simulink model "MCLV2_dsPIC33EP256MC506_externalOpAmp_CurrentLoop_FrSky"  (R2019a)
settings: Solver=FixedStepDiscrete  StartTime=0.0  StopTime=inf  FixedStep=.00005  RelTol=1e-3  EnableMultiTasking=on
values from neighbouring files (symbols this model uses):
  Imax = Inom    (= 4.3)    [DCMotorParameters.m]
  Imin = -Inom    (= -4.3)    [DCMotorParameters.m]
  Ke = place(Ae,Be,Elec_desired_poles)    [DCMotorParameters.m]
  Km = place(Am,Bm,Desired_mecha_pole)    [DCMotorParameters.m]
  Ommax = Omnom    (= 350)    [DCMotorParameters.m]
  Ommin = -Omnom    (= -350)    [DCMotorParameters.m]
  Ts = 0.5e-4    (= 5e-05)    [DCMotorParameters.m]
  TsMeca = 0.002    [DCMotorParameters.m]
  Vmax = Vdc    (= 24)    [DCMotorParameters.m]
  Vmin = -Vdc    (= -24)    [DCMotorParameters.m]
undefined symbols (not defined in the file or in its folder): A4, A8, B5, B6, C10, C5, C6, D5, DiscIntNeverNeededParam, F0, F1, Max, ms, NumBits1, NumBits2, P20, P24, P37, P53, P54, P97, Pin, PWMmax, Resol, us
libraries: simulink x26, MCHP_Blockset x25, UxV_Blockset x4
(part 2 of 2)

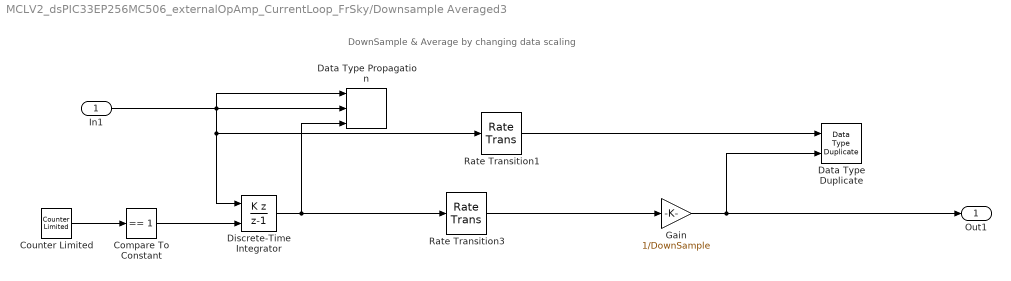
== system MCLV2_dsPIC33EP256MC506_externalOpAmp_CurrentLoop_FrSky/Downsample Averaged3 ==
  note: DownSample & Average by changing data scaling
  In1 : Inport
  Compare To Constant : simulink/Logic and Bit Operations/Compare To Constant  relop===  const=1  OutDataTypeStr=boolean
  Counter Limited : simulink/Sources/Counter Limited  uplimit=DownSample-1  tsamp=-1
  Data Type Duplicate : DataTypeDuplicate
  Data Type Propagation : simulink/Signal Attributes/Data Type Propagation  PropDataType=fixdt(1, 16)  IfRefDouble=double  IfRefSingle=single  IsSigned=IsSigned1 or IsSigned2  NumBitsBase=NumBits1+NumBits2  NumBitsMult=1  NumBitsAdd=0  NumBitsAllowFinal=1:128  PropScaling=2^-10  ValuesUsedBestPrec=[5 -7]  SlopeBase=Slope1  SlopeMult=1  SlopeAdd=0  BiasBase=Bias1  BiasMult=1  BiasAdd=0
      settings: SourceProductName=Simulink  SourceProductBaseCode=SL
  Discrete-Time Integrator : DiscreteIntegrator  IntegratorMethod=Accumulation: Backward Euler  gainval=1  ExternalReset=sampled level  SampleTime=-1  OutDataTypeStr=Inherit: Inherit via back propagation  ICPrevOutput=DiscIntNeverNeededParam  ICPrevScaledInput=DiscIntNeverNeededParam
  Gain : Gain  Gain=1/DownSample  OutDataTypeStr=Inherit: Inherit via back propagation
  Rate Transition1 : RateTransition  Deterministic=off  OutPortSampleTime=[InputSampleTime * DownSample]
  Rate Transition3 : RateTransition  OutPortSampleTime=[InputSampleTime * DownSample]
  Out1 : Outport
  wires:
  Rate Transition3/1 -> Gain/1
  In1/1 -> Discrete-Time Integrator/1, Rate Transition1/1, Data Type Propagation/2, Data Type Propagation/1
  Compare To Constant/1 -> Discrete-Time Integrator/2
  Discrete-Time Integrator/1 -> Data Type Propagation/3, Rate Transition3/1
  Counter Limited/1 -> Compare To Constant/1
  Gain/1 -> Data Type Duplicate/2, Out1/1
  Rate Transition1/1 -> Data Type Duplicate/1

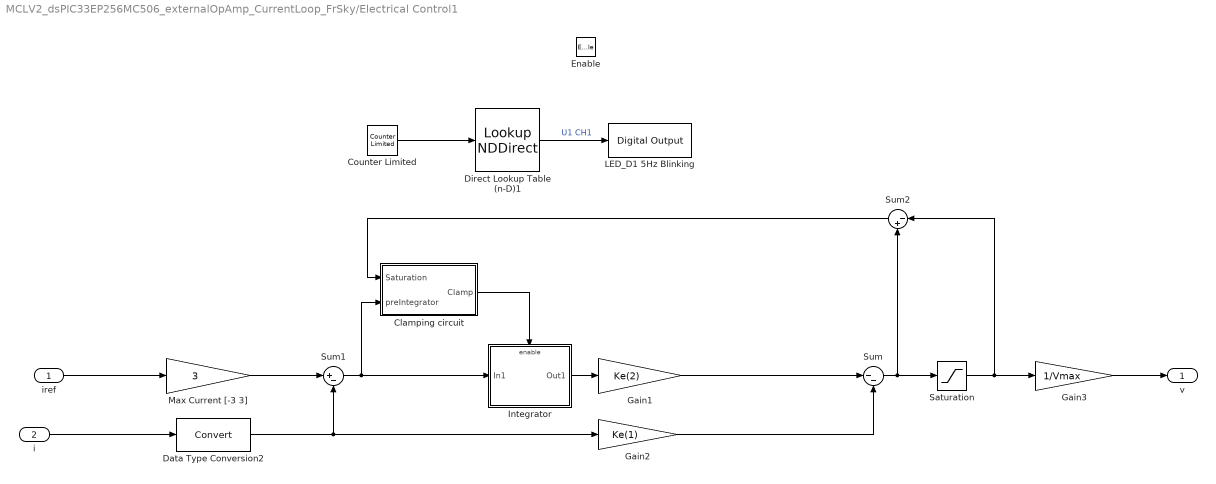
== system MCLV2_dsPIC33EP256MC506_externalOpAmp_CurrentLoop_FrSky/Electrical Control1 ==
  iref : Inport
  i : Inport  Port=2
  Enable : EnablePort  StatesWhenEnabling=reset
  Clamping circuit : Subsystem
  Counter Limited : simulink/Sources/Counter Limited  uplimit=9  tsamp=.1
  Data Type Conversion2 : DataTypeConversion  SaturateOnIntegerOverflow=on
  Direct Lookup Table (n-D)1 : LookupNDDirect  NumberOfTableDimensions=1  Table=[1 0 0 0 0 0 0 0 0 0]  TableDataTypeStr=boolean
  Gain1 : Gain  Gain=Ke(2)  OutMin=[2*Vmin]  OutMax=[2*Vmax]  OutDataTypeStr=fixdt(1,16)
  Gain2 : Gain  Gain=Ke(1)  OutMin=[2*Vmin]  OutMax=[2*Vmax]  OutDataTypeStr=fixdt(1,16)
  Gain3 : Gain  Gain=1/Vmax  OutDataTypeStr=fixdt(1,16,15)  SaturateOnIntegerOverflow=on
  Integrator : Subsystem
  LED_D1 5Hz Blinking : MCHP_Blockset/Digital IO/Digital Output  PORT=Dynamic Options  PORT_TXT="D   [ 5  6  8 ]"  PIN=6  PACK=off  SIMULTANEOUS=off  READPREVIOUS=off  ORDERING=None  SampleTime=-1  MCHP_MASTERLINK=MCLV2_dsPIC33EP256MC506_externalOpAmp_CurrentLoop_FrSky/Microchip Master
      settings: SourceProductName=MPLAB Device Blocks for Simulink
  Max Current [-3 3] : Gain  Gain=3  OutMin=-3  OutMax=3  OutDataTypeStr=fixdt(1,16)
  Saturation : Saturate  UpperLimit=Vmax  LowerLimit=Vmin
  Sum : Sum  Inputs=|--  SaturateOnIntegerOverflow=on
  Sum1 : Sum  Inputs=|+-  OutMin=[2*Imin]  OutMax=[2*Imax]  OutDataTypeStr=fixdt(1,16)  SaturateOnIntegerOverflow=on
  Sum2 : Sum  Inputs=|-+  OutDataTypeStr=Inherit: Same as accumulator
  v : Outport
  wires:
  iref/1 -> Max Current [-3 3]/1
  i/1 -> Data Type Conversion2/1
  Gain1/1 -> Sum/1
  Gain2/1 -> Sum/2
  Saturation/1 -> Sum2/1, Gain3/1
  Sum1/1 -> Integrator/1(In1), Clamping circuit/2(preIntegrator)
  Integrator/1(Out1) -> Gain1/1
  Clamping circuit/1(Clamp) -> Integrator/Enable
  Sum/1 -> Saturation/1, Sum2/2
  Sum2/1 -> Clamping circuit/1(Saturation)
  Data Type Conversion2/1 -> Gain2/1, Sum1/2
  Gain3/1 -> v/1
  Max Current [-3 3]/1 -> Sum1/1
  Direct Lookup Table (n-D)1/1 -> LED_D1 5Hz Blinking/1  "U1 CH1"
  Counter Limited/1 -> Direct Lookup Table (n-D)1/1

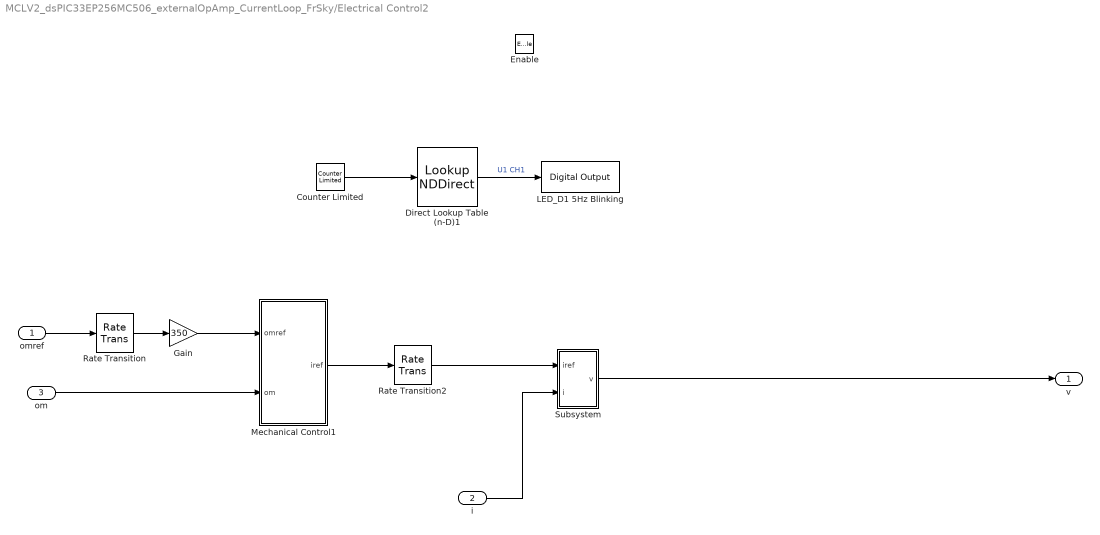
== system MCLV2_dsPIC33EP256MC506_externalOpAmp_CurrentLoop_FrSky/Electrical Control2 ==
  omref : Inport
  i : Inport  Port=2
  om : Inport  Port=3
  Enable : EnablePort  StatesWhenEnabling=reset
  Counter Limited : simulink/Sources/Counter Limited  uplimit=9  tsamp=.1
  Direct Lookup Table (n-D)1 : LookupNDDirect  NumberOfTableDimensions=1  Table=[1 0 1 0 0 0 0 0 0 0]  TableDataTypeStr=boolean
  Gain : Gain  Gain=350  OutDataTypeStr=Inherit: Inherit via back propagation
  LED_D1 5Hz Blinking : MCHP_Blockset/Digital IO/Digital Output  PORT=Dynamic Options  PORT_TXT="D   [ 5  6  8 ]"  PIN=6  PACK=off  SIMULTANEOUS=off  READPREVIOUS=off  ORDERING=None  SampleTime=-1  MCHP_MASTERLINK=MCLV2_dsPIC33EP256MC506_externalOpAmp_CurrentLoop_FrSky/Microchip Master
      settings: SourceProductName=MPLAB Device Blocks for Simulink
  Mechanical Control1 : Subsystem
  Rate Transition : RateTransition  Deterministic=off
  Rate Transition2 : RateTransition  Deterministic=off
  Subsystem : Subsystem
  v : Outport
  wires:
  i/1 -> Subsystem/2(i)
  Subsystem/1(v) -> v/1
  Mechanical Control1/1(iref) -> Rate Transition2/1
  Rate Transition2/1 -> Subsystem/1(iref)
  omref/1 -> Rate Transition/1
  Gain/1 -> Mechanical Control1/1(omref)
  Rate Transition/1 -> Gain/1
  om/1 -> Mechanical Control1/2(om)
  Direct Lookup Table (n-D)1/1 -> LED_D1 5Hz Blinking/1  "U1 CH1"
  Counter Limited/1 -> Direct Lookup Table (n-D)1/1

== system MCLV2_dsPIC33EP256MC506_externalOpAmp_CurrentLoop_FrSky/From Pot ==
  In1 : Inport
  Enable : EnablePort
  Cast5 : DataTypeConversion  OutDataTypeStr=boolean
  Counter Free-Running : simulink/Sources/Counter Free-Running  NumBits=1  tsamp=.1
  Gain : Gain  OutDataTypeStr=fixdt(1,16,15)
  LED_D1 5Hz Blinking : MCHP_Blockset/Digital IO/Digital Output  PORT=Dynamic Options  PORT_TXT="D   [ 5  6  8 ]"  PIN=6  PACK=off  SIMULTANEOUS=off  READPREVIOUS=off  ORDERING=None  SampleTime=-1  MCHP_MASTERLINK=MCLV2_dsPIC33EP256MC506_externalOpAmp_CurrentLoop_FrSky/Microchip Master
      settings: SourceProductName=MPLAB Device Blocks for Simulink
  Out1 : Outport
  wires:
  In1/1 -> Gain/1
  Gain/1 -> Out1/1  "Duty Cycle"
  Cast5/1 -> LED_D1 5Hz Blinking/1  "U1 CH1"
  Counter Free-Running/1 -> Cast5/1

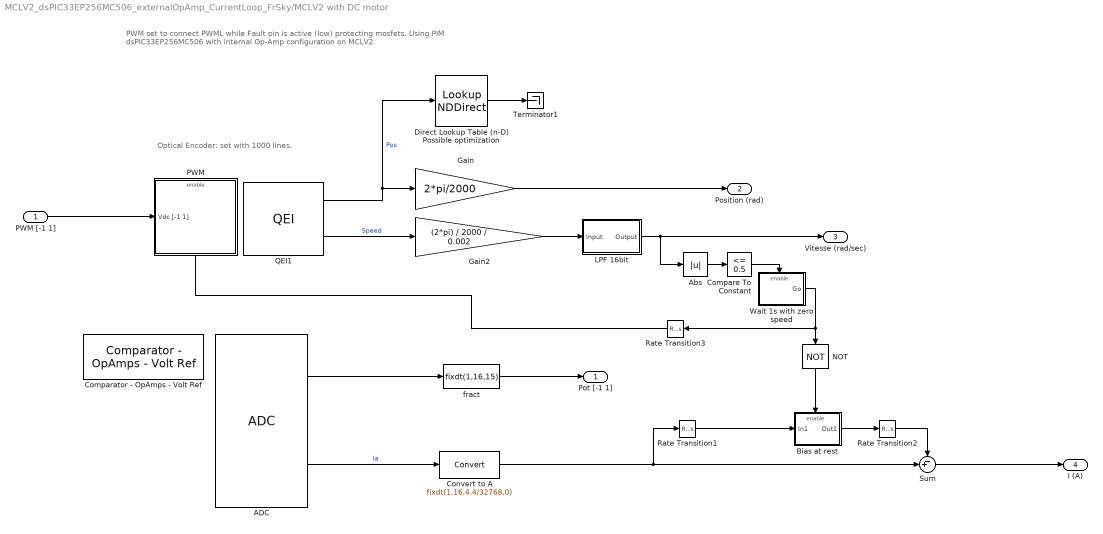
== system MCLV2_dsPIC33EP256MC506_externalOpAmp_CurrentLoop_FrSky/MCLV2 with DC motor ==
  note: PWM set to connect PWML while Fault pin is active (low) protecting mosfets.
      | Using PIM dsPIC33EP256MC506 with internal Op-Amp configuration on MCLV2
  note: Optical Encoder: set with 1000 lines.
  PWM [-1 1] : Inport
  ADC : MCHP_Blockset/Analog IO/ADC  Priority=5  ADC_REF=1  Mode=10 bits (allows exact simultaneous sampling)  FORM="sddd dddd dddd 0000  ==> Signed fractional"  ADC_R="< 5    kOhm"  nSAMPLECHANNELS=CH0 : CH1  nSAMPLECHANNELS_12bits=CH0 only  SIMULTANEOUS=Simultaneously on all Channels  ADxCSS=[13]  MUXA_CH0N=off  MUXA_CH123=Dynamic Options  MUXA_CH123_TXT=OA2 : AN1 : AN2  MUXB_CH0=AN1  MUXB_CH0N=on  MUXB_CH123=Dynamic Options  MUXB_CH123_TXT=OA2 : AN1 : AN2  SequenceRepeat=1  SequenceTiming=are done as fast as possible ; triggered by user define source  SSRC_SSRCG=Dynamic Options  SSRC_SSRCG_TXT=6  Update_BlockOutput=After each trig and conversion sequence  Trig_TimeStep=with each update of the ADC block output  ADC_DMA_CHANNEL=Use Interrupt instead of DMA  SampleTime=5e-05  Info=Total Time for Sample & Conversion : 2.4e-06s including 3.4286e-07s (x 1) sample time.  MCHP_PORT={Analog Input 0}{AN0}15:2:A0;{Analog Input 13}{AN13}15:2:E13;  MCHP_MASTERLINK=MCLV2_dsPIC33EP256MC506_externalOpAmp_CurrentLoop_FrSky/Microchip Master  ADC_TIMING=[2.4000000000000003149e-06]
      settings: SourceProductName=MPLAB Device Blocks for Simulink
  Abs : Abs
  Bias at rest : Subsystem  TreatAsAtomicUnit=on
  Comparator - OpAmps - Volt Ref : MCHP_Blockset/Analog IO/Comparator - OpAmps - Volt Ref  MCHP_params=s.CVR1OE=0;s.CVR2OE=0;s.VREFSEL=0;s.RLaddle=reshape([1 1],1,2);s.AVdd=reshape({ '3.3','3.3'},1,2);s.AVss=reshape({ '0','0'},1,2);s.CVRSS=reshape([0 0],1,2);s.CON_OPMODE_CPOL=reshape([0 3 0 0 0],1,5);s.OutputPort_COE_RP=reshape({ 'B1 / Pin[16] / OA1OUT / AN3 / OA1OUT','A0 / Pin[13] / OA2OUT / AN0 / OA2OUT','C0 / Pin[21] / OA3OUT / AN6 / OA3OUT','None','None'},1,5);s.InputP_CREF=reshape([0 0 0 0 0],1,5);s.InputN_CCH=reshape([0 0 0 0 0],1,5);s.Trigger_EventInterrupt_EVPOL=reshape([0 0 0 0 0],1,5);s.BlockOutputEvent=reshape([0 0 0 0 0],1,5);s.BlockOutputState=reshape([0 0 0 0 0],1,5);s.IntPriority=5;s.FilterFreq=reshape([1e+10 1e+10 1e+10 1e+10 1e+10],1,5);s.Blanking=reshape([1 1 1 1 1],1,5);s.BlankingSignal=reshape({ ' - ',' - ',' - ',' - ',' - ',' - ',' - ',' - ',' - ',' - ',' - ',' - ',' - ',' - ',' - '},3,5);s.BlankingTruthTable=reshape([-1 -1 -1 -1 -1 -1 -1 -1 -1 -1 -1 -1 -1 -1 -1 -1 -1 -1 -1 -1 -1 -1 -1 -1 -1 -1 -1 -1 -1 -1 -1 -1 -1 -1 -1 -1 -1 -1 -1 -1 -1 -1 -1 -1 -1 -1 -1 -1 -1 -1 -1 -1 -1 -1 -1 -1 -1 -1 -1 -1 -1 -1 -1 -1 -1 -1 -1 -1 -1 -1 -1 -1 -1 -1 -1 -1 -1 -1 -1 -1 -1 -1 -1 -1 -1 -1 -1 -1 -1 -1 -1 -1 -1 -1 -1 -1 -1 -1 -1 -1 -1 -1 -1 -1 -1 -1 -1 -1 -1 -1 -1 -1 -1 -1 -1 -1 -1 -1 -1 -1 -1 -1 -1 -1 -1 -1 -1 -1 -1 -1 -1 -1 -1 -1 -1 -1 -1 -1 -1 -1 -1 -1 -1 -1 -1 -1 -1 -1 -1 -1 -1 -1 -1 -1 -1 -1 -1 -1 -1 -1 -1 -1 -1 -1 -1 -1 -1 -1 -1 -1 -1 -1 -1 -1 -1 -1 -1 -1 -1 -1 -1 -1 -1 -1 -1 -1 -1 -1 -1 -1 -1 -1 -1 -1 -1 -1 -1 -1 -1 -1 -1 -1 -1 -1 -1 -1 -1 -1 -1 -1 -1 -1 -1 -1 -1 -1 -1 -1 -1 -1 -1 -1 -1 -1 -1 -1 -1 -1 -1 -1 -1 -1 -1 -1 -1 -1 -1 -1 -1 -1],16 ,3 ,5);  S_INPUT="[5  5]"  S_OUTPUT=[5]  S_INPUT_Size="[2  2]"  S_OUTPUT_Size=[4]  SampleTime=-1  MCHP_MASTERLINK=MCLV2_dsPIC33EP256MC506_externalOpAmp_CurrentLoop_FrSky/Microchip Master  MCHP_PORT={Op-Amp Output 2}{OA2(out)}14:2:A0;{Op-Amp2 V+}{OA2 V+}14:2:A1;{Op-Amp2 V-}{OA2 V-}14:2:B0;  ORDERING=0
      settings: SourceProductName=MPLAB Device Blocks for Simulink
  Compare To Constant : simulink/Logic and Bit Operations/Compare To Constant  relop=<=  const=0.5  OutDataTypeStr=boolean
  Convert to A : DataTypeConversion  OutDataTypeStr=fixdt(1,16,4.4/32768,0)  ConvertRealWorld=Stored Integer (SI)
  Direct Lookup Table (n-D) Possible optimization : LookupNDDirect  NumberOfTableDimensions=1  Table=[0:(1000-1)]*2*pi/1000  TableDataTypeStr=fixdt(1,16,5)
      settings: LockScale=on
  Gain : Gain  Gain=2*pi/2000  OutDataTypeStr=fixdt(1,16,5)
  Gain2 : Gain  Gain=(2*pi) / 2000 / 0.002  OutDataTypeStr=fixdt(1,16,5)  LockScale=on
  "LPF 16bit " : Subsystem  Tag=FilterWizardSubSystem
      settings: ErrorFcn=dspFilterRealizedInBasicElemsAlgLoopErrFcnCallback
  NOT : Logic  Operator=NOT  IconShape=distinctive  AllPortsSameDT=off  OutDataTypeStr=boolean
  PWM : Subsystem
  QEI1 : MCHP_Blockset/QEI/QEI  QEI_REF=1  QEI_MODE=Quadrature Encoder  QEI_x2mode=off  QEI_PulseCountDir=Down  PIN_QEA=Dynamic Options  PIN_QEA_TXT=A8 / P24 / Pin[31]  PIN_QEB=Dynamic Options  PIN_QEB_TXT=C6 / P54 / Pin[50]  SWPAB=off  QEAPOL=off  QEBPOL=off  SampleTime=.002  PIN_CCMP=Dynamic Options  PIN_CCMP_TXT=A4 / P20 / Pin[33]  MCHP_PORT={QEI1 A}{QEIA1}5:0:P24;{QEI1 B}{QEIB1}5:0:P54;  MCHP_MASTERLINK=MCLV2_dsPIC33EP256MC506_externalOpAmp_CurrentLoop_FrSky/Microchip Master  INDXxCNT_Output=is not an output  POSxCNT_Output=is a 16 bits unsigned block output  RESET_Input=off  PIMOD_mode=position is cyclique between user defined boundaries  PIMOD_modeB=Never reset position  PIMOD_reset=on next INDEX event  PIN_INDEX=Dynamic Options  PIN_INDEX_TXT=A4 / P20 / Pin[33]  IMV=QEA = 1 and QEB = 0  IMV_x2=QEA = 1  PIN_HOME=Dynamic Options  PIN_HOME_TXT=A4 / P20 / Pin[33]  QEIxLEC_GEC=[0 1999]  QEIxIC=0  PCIIRQ=off  IDXPOL=off  HOMPOL=on  VELxCNT_Output=is a 16 bits signed block output  INTxHLD_Output=is not an output  MaxPeriod=1e-3  FILTREN=on  QFDIV_popup=Dynamic Options  QFDIV_popup_TXT=729.17 kHz  FILTER_CutOffFreq=100e3  QEI_IntPri=5
      settings: SourceProductName=MPLAB Device Blocks for Simulink
  Rate Transition1 : RateTransition  Deterministic=off  OutPortSampleTime=.002
  Rate Transition2 : RateTransition  Deterministic=off
  Rate Transition3 : RateTransition  Deterministic=off
  Sum : Sum  Inputs=-+|  OutDataTypeStr=Inherit: Inherit via back propagation  SaturateOnIntegerOverflow=on  InputSameDT=on
  Terminator1 : Terminator
  Wait 1s with zero speed : Subsystem  TreatAsAtomicUnit=on
  fract : DataTypeConversion  OutDataTypeStr=fixdt(1,16,15)  ConvertRealWorld=Stored Integer (SI)
  Pot [-1 1] : Outport
  Position (rad) : Outport  Port=2
  Vitesse (rad/sec) : Outport  Port=3
  I (A) : Outport  Port=4
  wires:
  Abs/1 -> Compare To Constant/1
  Rate Transition3/1 -> PWM/Enable
  Compare To Constant/1 -> Wait 1s with zero speed/Enable
  Wait 1s with zero speed/1(Go) -> NOT/1, Rate Transition3/1
  PWM [-1 1]/1 -> PWM/1(Vdc [-1 1])
  NOT/1 -> Bias at rest/Enable
  Rate Transition2/1 -> Sum/1
  Rate Transition1/1 -> Bias at rest/1(In1)
  Bias at rest/1(Out1) -> Rate Transition2/1
  Sum/1 -> I (A)/1
  ADC/2 -> Convert to A/1  "Ia"
  Convert to A/1 -> Rate Transition1/1, Sum/2
  "LPF 16bit "/1(Output) -> Abs/1, Vitesse (rad/sec)/1
  Gain2/1 -> "LPF 16bit "/1(Input)
  Gain/1 -> Position (rad)/1
  fract/1 -> Pot [-1 1]/1
  QEI1/1 -> Gain/1, Direct Lookup Table (n-D) Possible optimization/1  "Pos"
  ADC/1 -> fract/1
  QEI1/2 -> Gain2/1  "Speed"
  Direct Lookup Table (n-D) Possible optimization/1 -> Terminator1/1

== system MCLV2_dsPIC33EP256MC506_externalOpAmp_CurrentLoop_FrSky/Steps Large ==
  Enable : EnablePort  StatesWhenEnabling=reset
  Constant : Constant  Value=0  OutDataTypeStr=Inherit: Inherit via back propagation
  Counter Limited : simulink/Sources/Counter Limited  uplimit=9  tsamp=.1
  Direct Lookup Table (n-D)1 : LookupNDDirect  NumberOfTableDimensions=1  Table=[1 0 1 0 1 0 0 0 0 0]  TableDataTypeStr=boolean
  LED_D1 5Hz Blinking : MCHP_Blockset/Digital IO/Digital Output  PORT=Dynamic Options  PORT_TXT="D   [ 5  6  8 ]"  PIN=6  PACK=off  SIMULTANEOUS=off  READPREVIOUS=off  ORDERING=None  SampleTime=-1  MCHP_MASTERLINK=MCLV2_dsPIC33EP256MC506_externalOpAmp_CurrentLoop_FrSky/Microchip Master
      settings: SourceProductName=MPLAB Device Blocks for Simulink
  Out1 : Outport
  wires:
  Constant/1 -> Out1/1
  Counter Limited/1 -> Direct Lookup Table (n-D)1/1
  Direct Lookup Table (n-D)1/1 -> LED_D1 5Hz Blinking/1  "U1 CH1"

== system MCLV2_dsPIC33EP256MC506_externalOpAmp_CurrentLoop_FrSky/Timing Analysis ==
  note: Task 1 -> RB5 (PGD2)
      | Task 2 -> RB6 (PGC2)
      | Task 3 -> RF0 (HALL C)
      | Load: -> RC10  (HOME)
      | Overload -> LED 1
  MCU Load : MCHP_Blockset/Profiling/MCU Load  MCULoadPin=Dynamic Options  MCULoadPin_TXT=C10 / Pin[45]  MCULoadMeasure=off  TIMER_Resolution=Dynamic Options  TIMER_Resolution_TXT="Resol: 0.1143(us)  -  Max: 7.49(ms)"  MCHP_PORT={MCU Load Pin}{MCU_Load}0:1:C10;  MCHP_TIMER_REQUEST={MCU_Load}{MCU_Load}21:5:0:0:[]:524288;  MCHP_TIMER_RESULT=[1 65535 ]  MCHP_MASTERLINK=MCLV2_dsPIC33EP256MC506_externalOpAmp_CurrentLoop/Microchip Master  MCHP_COMPILED_INFO=CompiledSampleTime= [Inf Inf ];CompiledInportDataTypes=[ ];CompiledInportDataWidth=[];  Info="Timer 1:  Resol: 114.2857143(ns)  -  Max: 7.48983(ms)"  SampleTime=-1
      settings: SourceProductName=MPLAB Device Blocks for Simulink
  MCU Overload : MCHP_Blockset/Profiling/MCU Overload  MCUOverloadBlockOutput=off  MCUOverLoadPin=Dynamic Options  MCUOverLoadPin_TXT=D5 / Pin[53]  MCHP_PORT={OverLoad Pin}{OverLoad}0:1:D5;  MCHP_MASTERLINK=MCLV2_dsPIC33EP256MC506_externalOpAmp_CurrentLoop/Microchip Master  SampleTime=.1
      settings: SourceProductName=MPLAB Device Blocks for Simulink
  Tasks State : MCHP_Blockset/Profiling/Tasks State  TasksPin=[B5 B6 F0]  MCHP_PORT={Task D1 Running}{Task D1}15:1:B5;{Task D2 Running}{Task D2}15:1:B6;{Task D3 Running}{Task D3}15:1:F0;  MCHP_MASTERLINK=MCLV2_dsPIC33EP256MC506_externalOpAmp_CurrentLoop/Microchip Master
      settings: SourceProductName=MPLAB Device Blocks for Simulink

== system MCLV2_dsPIC33EP256MC506_externalOpAmp_CurrentLoop_FrSky/Toggle (4 states) ==
  In1 : Inport
  Bitwise Operator : simulink/Logic and Bit Operations/Bitwise Operator  logicop=AND  UseBitMask=on  BitMask=7  BitMaskRealWorld=Stored Integer
  Delay : Delay  DelayLength=1  InitialCondition=0
  Detect Increase : simulink/Logic and Bit Operations/Detect Increase  vinit=1  OutDataTypeStr=boolean
  Sum : Sum  AccumDataTypeStr=uint16  OutDataTypeStr=uint16
  Out1 : Outport
  wires:
  Delay/1 -> Sum/2
  Sum/1 -> Bitwise Operator/1
  Detect Increase/1 -> Sum/1
  In1/1 -> Detect Increase/1
  Bitwise Operator/1 -> Out1/1, Delay/1

== system MCLV2_dsPIC33EP256MC506_externalOpAmp_CurrentLoop_FrSky/Electrical Control1/Clamping circuit ==
  note: The clamping enable or disable the integral action.
  Saturation : Inport  DisableCoverage=on
  preIntegrator : Inport  DisableCoverage=on  Port=2
  Compare To Zero1 : simulink/Logic and Bit Operations/Compare To Zero  relop=<=  OutDataTypeStr=boolean
  Delay : Delay  DelayLength=1  InitialCondition=0
  Multiply : Product
  Clamp : Outport  DisableCoverage=on
  wires:
  Compare To Zero1/1 -> Clamp/1
  preIntegrator/1 -> Multiply/2
  Multiply/1 -> Compare To Zero1/1
  Saturation/1 -> Delay/1
  Delay/1 -> Multiply/1

== system MCLV2_dsPIC33EP256MC506_externalOpAmp_CurrentLoop_FrSky/Electrical Control1/Integrator ==
  In1 : Inport
  Enable : EnablePort
  Discrete-Time Integrator : DiscreteIntegrator  SampleTime=Ts  OutMin=[2*Imin]  OutMax=[2*Imax]  OutDataTypeStr=fixdt(1,32)  ICPrevOutput=DiscIntNeverNeededParam  ICPrevScaledInput=DiscIntNeverNeededParam
  Out1 : Outport
  wires:
  Discrete-Time Integrator/1 -> Out1/1
  In1/1 -> Discrete-Time Integrator/1

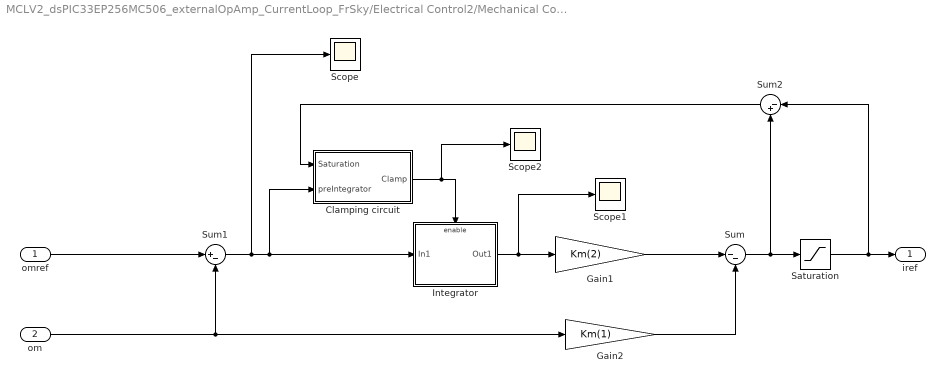
== system MCLV2_dsPIC33EP256MC506_externalOpAmp_CurrentLoop_FrSky/Electrical Control2/Mechanical Control1 ==
  omref : Inport  OutMin=[Ommin]  OutMax=[Ommax]  OutDataTypeStr=fixdt(1,16)
  om : Inport  Port=2
  Clamping circuit : Subsystem
  Gain1 : Gain  Gain=Km(2)  OutMin=[-2*Imax]  OutMax=[2*Imax]  OutDataTypeStr=fixdt(1,16)
  Gain2 : Gain  Gain=Km(1)  OutMin=[-2*Imax]  OutMax=[2*Imax]  OutDataTypeStr=fixdt(1,16)
  Integrator : Subsystem
  Saturation : Saturate  UpperLimit=Imax  LowerLimit=Imin
  Scope : Scope
  Scope1 : Scope
  Scope2 : Scope
  Sum : Sum  Inputs=|--  SaturateOnIntegerOverflow=on
  Sum1 : Sum  Inputs=|+-  OutMin=[2*Ommin]  OutMax=[2*Ommax]  OutDataTypeStr=fixdt(1,16)  SaturateOnIntegerOverflow=on
  Sum2 : Sum  Inputs=|-+  OutDataTypeStr=Inherit: Same as accumulator
  iref : Outport
  wires:
  Gain1/1 -> Sum/1
  Sum1/1 -> Scope/1, Clamping circuit/2(preIntegrator), Integrator/1(In1)
  omref/1 -> Sum1/1
  Gain2/1 -> Sum/2
  om/1 -> Gain2/1, Sum1/2
  Sum2/1 -> Clamping circuit/1(Saturation)
  Sum/1 -> Sum2/2, Saturation/1
  Clamping circuit/1(Clamp) -> Scope2/1, Integrator/Enable
  Saturation/1 -> Sum2/1, iref/1
  Integrator/1(Out1) -> Scope1/1, Gain1/1

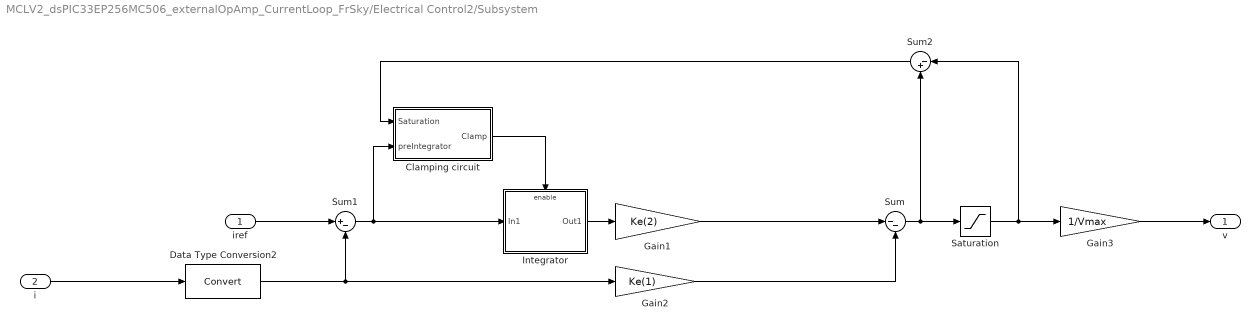
== system MCLV2_dsPIC33EP256MC506_externalOpAmp_CurrentLoop_FrSky/Electrical Control2/Subsystem ==
  iref : Inport
  i : Inport  Port=2
  Clamping circuit : Subsystem
  Data Type Conversion2 : DataTypeConversion  SaturateOnIntegerOverflow=on
  Gain1 : Gain  Gain=Ke(2)  OutMin=[2*Vmin]  OutMax=[2*Vmax]  OutDataTypeStr=fixdt(1,16)
  Gain2 : Gain  Gain=Ke(1)  OutMin=[2*Vmin]  OutMax=[2*Vmax]  OutDataTypeStr=fixdt(1,16)
  Gain3 : Gain  Gain=1/Vmax  OutDataTypeStr=fixdt(1,16,15)  SaturateOnIntegerOverflow=on
  Integrator : Subsystem
  Saturation : Saturate  UpperLimit=Vmax  LowerLimit=Vmin
  Sum : Sum  Inputs=|--  SaturateOnIntegerOverflow=on
  Sum1 : Sum  Inputs=|+-  OutMin=[2*Imin]  OutMax=[2*Imax]  OutDataTypeStr=fixdt(1,16)  SaturateOnIntegerOverflow=on
  Sum2 : Sum  Inputs=|-+  OutDataTypeStr=Inherit: Same as accumulator
  v : Outport
  wires:
  i/1 -> Data Type Conversion2/1
  Saturation/1 -> Gain3/1, Sum2/1
  Sum/1 -> Sum2/2, Saturation/1
  Gain2/1 -> Sum/2
  Gain1/1 -> Sum/1
  Data Type Conversion2/1 -> Sum1/2, Gain2/1
  Sum1/1 -> Clamping circuit/2(preIntegrator), Integrator/1(In1)
  iref/1 -> Sum1/1
  Clamping circuit/1(Clamp) -> Integrator/Enable
  Sum2/1 -> Clamping circuit/1(Saturation)
  Gain3/1 -> v/1
  Integrator/1(Out1) -> Gain1/1

== system MCLV2_dsPIC33EP256MC506_externalOpAmp_CurrentLoop_FrSky/MCLV2 with DC motor/Bias at rest ==
  In1 : Inport
  Enable : EnablePort
  LPF_3Hz : Subsystem  Tag=FilterWizardSubSystem
      settings: ErrorFcn=dspFilterRealizedInBasicElemsAlgLoopErrFcnCallback
  Out1 : Outport  InitialOutput=0
  wires:
  LPF_3Hz/1(Output) -> Out1/1
  In1/1 -> LPF_3Hz/1(Input)

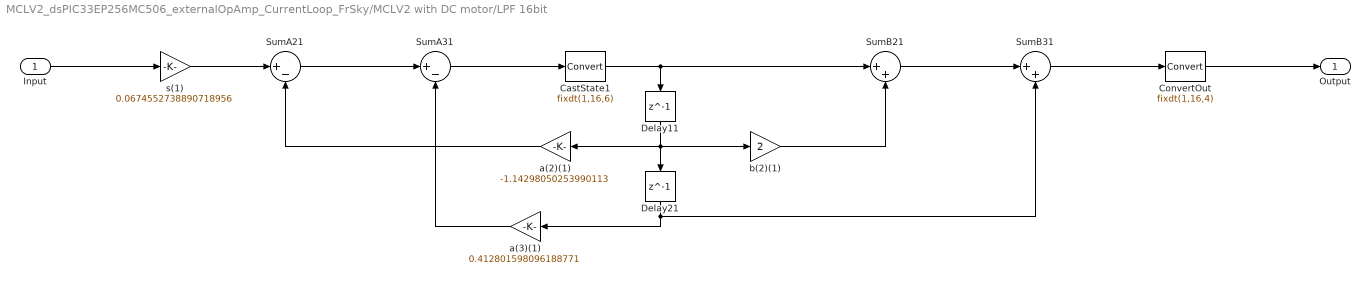
== system MCLV2_dsPIC33EP256MC506_externalOpAmp_CurrentLoop_FrSky/MCLV2 with DC motor/LPF 16bit  ==
  Input : Inport
  CastState1 : DataTypeConversion  OutDataTypeStr=fixdt(1,16,6)
  ConvertOut : DataTypeConversion  OutDataTypeStr=fixdt(1,16,4)
  Delay11 : Delay  DelayLength=1  InitialCondition=0
  Delay21 : Delay  DelayLength=1  InitialCondition=0
  SumA21 : Sum  Inputs=|+-  AccumDataTypeStr=fixdt(1,16,6)  OutDataTypeStr=fixdt(1,16,6)
  SumA31 : Sum  Inputs=|+-  AccumDataTypeStr=fixdt(1,16,6)  OutDataTypeStr=fixdt(1,16,6)
  SumB21 : Sum  Inputs=|++  AccumDataTypeStr=fixdt(1,16,5)  OutDataTypeStr=fixdt(1,16,5)
  SumB31 : Sum  Inputs=|++  AccumDataTypeStr=fixdt(1,16,4)  OutDataTypeStr=fixdt(1,16,4)
  a(2)(1) : Gain  Gain=-1.14298050253990113  ParamDataTypeStr=fixdt(1,16,14)  OutDataTypeStr=fixdt(1,16,6)
  a(3)(1) : Gain  Gain=0.412801598096188771  ParamDataTypeStr=fixdt(0,16,17)  OutDataTypeStr=fixdt(1,16,8)
  b(2)(1) : Gain  Gain=2  ParamDataTypeStr=fixdt(0,16,14)  OutDataTypeStr=fixdt(1,16,5)
  s(1) : Gain  Gain=0.0674552738890718956  ParamDataTypeStr=fixdt(0,16,19)  OutDataTypeStr=fixdt(1,16,8)
  Output : Outport
  wires:
  Input/1 -> s(1)/1
  ConvertOut/1 -> Output/1
  Delay21/1 -> SumB31/2, a(3)(1)/1
  a(3)(1)/1 -> SumA31/2
  b(2)(1)/1 -> SumB21/2
  Delay11/1 -> Delay21/1, b(2)(1)/1, a(2)(1)/1
  a(2)(1)/1 -> SumA21/2
  SumB31/1 -> ConvertOut/1
  SumB21/1 -> SumB31/1
  CastState1/1 -> Delay11/1, SumB21/1
  SumA31/1 -> CastState1/1
  SumA21/1 -> SumA31/1
  s(1)/1 -> SumA21/1

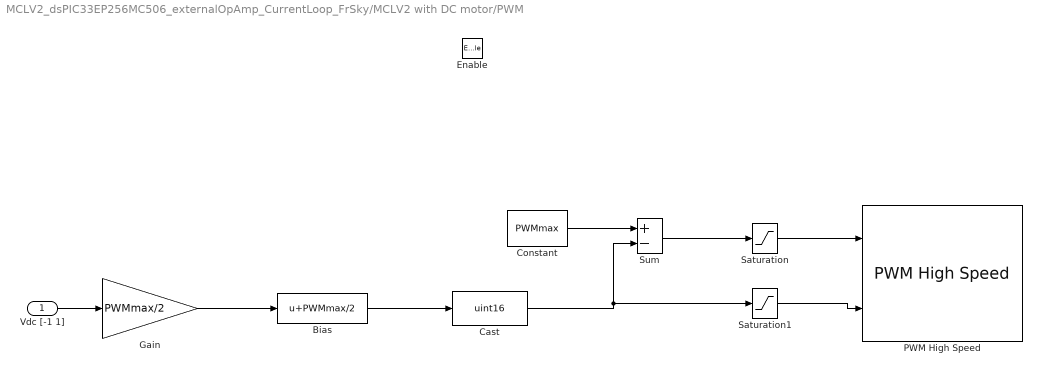
== system MCLV2_dsPIC33EP256MC506_externalOpAmp_CurrentLoop_FrSky/MCLV2 with DC motor/PWM ==
  Vdc [-1 1] : Inport
  Enable : EnablePort
  Bias : Bias  Bias=PWMmax/2
  Cast : DataTypeConversion  OutDataTypeStr=uint16
  Constant : Constant  Value=PWMmax  OutDataTypeStr=uint16
  Gain : Gain  Gain=PWMmax/2  OutDataTypeStr=fixdt(1,32,1)
  PWM High Speed : MCHP_Blockset/PWM IO/PWM High Speed  pop1=[1]  chk1="[1  1  1  0  0]"  chkHL1="[1  1  0  1  1  1  1  1 ; 1  1  0  1  1  1  1  1]"  maxP1={ '50e-6','0.001','0.001','0.001','0.001','0.001','0.001','0.001';'0.001','0.001','1e-06','0.001','0.001','0.001','0.001','0.001'}  InitP2={ '50e-6','.001','0.001','0.001','0.001','0.001','0.001','0.001';'0.001','0.001','0.001','0.001','0.001','0.001','0.001','0.001'}  chkP2="[0  1  0  1  1  1  1  1 ; 1  0  0  1  1  1  1  1]"  InitDC={ '50','50','50','50','50','50','50','50';'0.001','0.001','0.001','50','50','50','50','50'}  chkDC="[1  1  1  1  1  1  1  1 ; 0  0  0  1  1  1  1  1]"  InitPh={ '0','0','0','0.001','0.001','0.001','0.001','0.001';'0','0','0','0.001','0.001','0.001','0.001','0.001'}  chkPh="[0  0  0  1  1  1  1  1 ; 0  0  0  1  1  1  1  1]"  edSEvTrigx={ '120e-9','-1','-1','-1','-1','-1','-1','-1'}  chkSEvTrigx="[0  1  1  1  1  1  1  1]"  popFlt="[2  2  1  1  1  1  1  1]"  popFltPin="[20  20  20   4   4   4   4   4]"  popFltPinRp="[1  1  1  1  1  1  1]"  popFltActivH="[2  2  1  1  1  1  1  1]"  popFltForceH="[2  2  2  2  2  2  2  2]"  popFltForceL="[1  1  1  1  1  1  1  1]"  chkFltBlkOut="[0  0  0  0  0  0  0  0]"  popIndepFaultMode="[1  1  1  1  1  1  1  1]"  popCurEnabled="[1  1  1  1  1  1  1  1]"  popCurPin="[4  31   4   4   4   4   4   4]"  popCurActiveH="[1  1  1  1  1  1  1  1]"  popCurForceH="[2  1  2  1  1  1  1  1]"  popCurForceL="[2  1  2  1  1  1  1  1]"  ChkCurBlkOut="[0  0  0  0  0  0  0  0]"  ChkCurBlkOutTime="[0  0  1  0  0  0  0  0]"  popBLANKSEL="[1  1  1  1  1  1  1  1]"  popBPHHBPHL="[1  1  1  1  1  1  1  1]"  popBPLHBPLL="[1  1  1  1  1  1  1  1]"  popFLTLEBEN_CLLEBEN="[1  1  1  1  1  1  1  1]"  popPHR_PHF="[2  1  1  1  1  1  1  1]"  popPLR_PLF="[3  1  1  1  1  1  1  1]"  edLEB={ '100e-9','50e-9','150e-9','50e-9','50e-9','50e-9','50e-9','50e-9'}  popDT="[1  1  1  3  3  3  3  3]"  edDTRx={ '0.02','1e-05','0.001','1e-05','1e-05','1e-05','1e-05','1e-05'}  edAltDTRx={ '0.5e-6','0.5e-6','0.5e-6','1e-05','1e-05','1e-05','1e-05','1e-05'}  S_INPUT="[5  5  5]"  S_INPUT_Size="[1  1  1]"  S_OUTPUT=[]  S_OUTPUT_Size=[]  S_DWORK_Type=[]  S_DWORK_Size=[]  ADC_VARTRIG={PWM Primary Special Event Trigger;6}  evalin_ws=PWMmax = 3499;PWM1max = 3499;PWM2max = 3499;  SampleTime=-1  ORDERING=None  MCHP_PORT={PWM1 Fault}{FLT32}4:0:B4;{PWM2 Fault}{FLT32}4:0:B4;{PWM1H}{PWM1H}4:4:B14;{PWM1L}{PWM1L}4:4:B15;{PWM2H}{PWM2H}4:4:B12;{PWM2L}{PWM2L}4:4:B13;  MCHP_MASTERLINK=MCLV2_dsPIC33EP256MC506_externalOpAmp_CurrentLoop_FrSky/Microchip Master  MCHP_VERSION=v3.39  Parameter50=0
      settings: SourceProductName=MPLAB Device Blocks for Simulink
  Saturation : Saturate  UpperLimit=PWMmax - (1e-6/50e-6)*PWMmax  LowerLimit=round( (0.5e-6/50e-6) *PWMmax )
  Saturation1 : Saturate  UpperLimit=PWMmax  LowerLimit=round( (0.5e-6/50e-6) *PWMmax )
  Sum : Sum  Inputs=+-  OutDataTypeStr=Inherit: Same as first input
  wires:
  Constant/1 -> Sum/1
  Vdc [-1 1]/1 -> Gain/1
  Saturation/1 -> PWM High Speed/1
  Bias/1 -> Cast/1
  Sum/1 -> Saturation/1
  Saturation1/1 -> PWM High Speed/2
  Cast/1 -> Saturation1/1, Sum/2
  Gain/1 -> Bias/1

== system MCLV2_dsPIC33EP256MC506_externalOpAmp_CurrentLoop_FrSky/MCLV2 with DC motor/Wait 1s with zero speed ==
  Enable : EnablePort
  "1s " : simulink/Logic and Bit Operations/Compare To Constant  relop=>=  const=500  OutDataTypeStr=boolean
  Constant : Constant  OutDataTypeStr=Inherit: Inherit via back propagation
  Discrete-Time Integrator : DiscreteIntegrator  IntegratorMethod=Accumulation: Forward Euler  gainval=1  SampleTime=-1  OutDataTypeStr=uint16  SaturateOnIntegerOverflow=on  ICPrevOutput=DiscIntNeverNeededParam  ICPrevScaledInput=DiscIntNeverNeededParam
  Go : Outport  InitialOutput=0
  wires:
  Discrete-Time Integrator/1 -> "1s "/1
  Constant/1 -> Discrete-Time Integrator/1
  "1s "/1 -> Go/1

== system MCLV2_dsPIC33EP256MC506_externalOpAmp_CurrentLoop_FrSky/Electrical Control2/Mechanical Control1/Clamping circuit ==
  note: La logique de clamping permet de bloquer l'entée de l'action intégrale.
      | Ainsi, si la sortie du controlleur est en dehors des limites imposés (saturée), alors l'action intégrale du correcteur est verrouyé (clamping).
      | L'action intégrale est verroullé si la sortie du correcteur (commande) est en dehors des saturations et que le signe de cette sortie est égale
      | à l'entrée du signal à intégrer.
  Saturation : Inport  DisableCoverage=on
  preIntegrator : Inport  DisableCoverage=on  Port=2
  Compare To Zero1 : simulink/Logic and Bit Operations/Compare To Zero  relop=<=  OutDataTypeStr=boolean
  Delay : Delay  DelayLength=1  InitialCondition=0  SampleTime=TsMeca
  Multiply : Product
  Clamp : Outport  DisableCoverage=on
  wires:
  Compare To Zero1/1 -> Clamp/1
  preIntegrator/1 -> Multiply/2
  Multiply/1 -> Compare To Zero1/1
  Saturation/1 -> Delay/1
  Delay/1 -> Multiply/1

== system MCLV2_dsPIC33EP256MC506_externalOpAmp_CurrentLoop_FrSky/Electrical Control2/Mechanical Control1/Integrator ==
  In1 : Inport
  Enable : EnablePort
  Discrete-Time Integrator : DiscreteIntegrator  SampleTime=TsMeca  OutMin=[2*Ommin]  OutMax=[2*Ommax]  OutDataTypeStr=fixdt(1,32)  ICPrevOutput=DiscIntNeverNeededParam  ICPrevScaledInput=DiscIntNeverNeededParam
  Out1 : Outport
  wires:
  Discrete-Time Integrator/1 -> Out1/1
  In1/1 -> Discrete-Time Integrator/1

== system MCLV2_dsPIC33EP256MC506_externalOpAmp_CurrentLoop_FrSky/Electrical Control2/Subsystem/Clamping circuit ==
  note: The clamping enable or disable the integral action.
  Saturation : Inport  DisableCoverage=on
  preIntegrator : Inport  DisableCoverage=on  Port=2
  Compare To Zero1 : simulink/Logic and Bit Operations/Compare To Zero  relop=<=  OutDataTypeStr=boolean
  Delay : Delay  DelayLength=1  InitialCondition=0
  Multiply : Product
  Clamp : Outport  DisableCoverage=on
  wires:
  Delay/1 -> Multiply/1
  Saturation/1 -> Delay/1
  Multiply/1 -> Compare To Zero1/1
  preIntegrator/1 -> Multiply/2
  Compare To Zero1/1 -> Clamp/1

== system MCLV2_dsPIC33EP256MC506_externalOpAmp_CurrentLoop_FrSky/Electrical Control2/Subsystem/Integrator ==
  In1 : Inport
  Enable : EnablePort
  Discrete-Time Integrator : DiscreteIntegrator  SampleTime=Ts  OutMin=[2*Imin]  OutMax=[2*Imax]  OutDataTypeStr=fixdt(1,32)  ICPrevOutput=DiscIntNeverNeededParam  ICPrevScaledInput=DiscIntNeverNeededParam
  Out1 : Outport
  wires:
  In1/1 -> Discrete-Time Integrator/1
  Discrete-Time Integrator/1 -> Out1/1

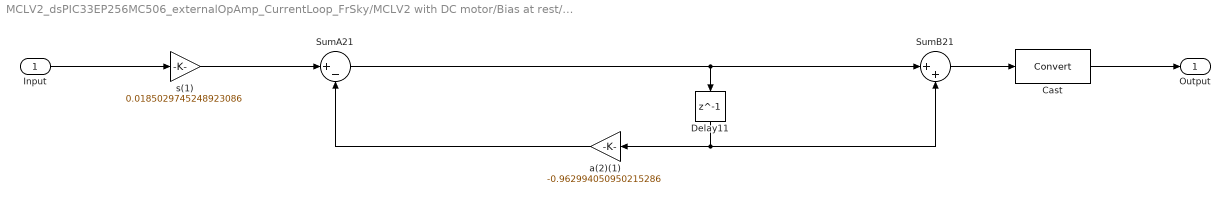
== system MCLV2_dsPIC33EP256MC506_externalOpAmp_CurrentLoop_FrSky/MCLV2 with DC motor/Bias at rest/LPF_3Hz ==
  Input : Inport
  Cast : DataTypeConversion
  Delay11 : Delay  DelayLength=1  InitialCondition=0
  SumA21 : Sum  Inputs=|+-  RndMeth=Convergent  SaturateOnIntegerOverflow=on  OutDataTypeStr=Inherit: Same as first input
  SumB21 : Sum  Inputs=|++  RndMeth=Simplest  SaturateOnIntegerOverflow=on  OutDataTypeStr=Inherit: Same as first input
  a(2)(1) : Gain  Gain=-0.962994050950215286  ParamDataTypeStr=fixdt(1,16,14)  RndMeth=Simplest  OutDataTypeStr=Inherit: Same as input
  s(1) : Gain  Gain=0.0185029745248923086  ParamDataTypeStr=fixdt(1,16,20)  OutDataTypeStr=fixdt(1,16,16)  RndMeth=Convergent  SaturateOnIntegerOverflow=on
  Output : Outport
  wires:
  Cast/1 -> Output/1
  Input/1 -> s(1)/1
  SumB21/1 -> Cast/1
  Delay11/1 -> SumB21/2, a(2)(1)/1
  a(2)(1)/1 -> SumA21/2
  SumA21/1 -> Delay11/1, SumB21/1
  s(1)/1 -> SumA21/1
